simulink model "Grid_forming_reproduction"  (R2023b)
settings: Solver=VariableStepAuto  StartTime=0.0  StopTime=30  RelTol=1e-3
PreLoadFcn:
  | Ts = 50e-6;
InitFcn:
  | load Grid_forming_reproduction_Init
  | Ts = 50e-6;
undefined symbols (not defined in the file or in its folder): DiscIntNeverNeededParam, find_system
libraries: spsThreePhaseVIMeasurementLib x6, spsabctodq0Lib x6, slpidlib x4, spsThreePhaseSeriesRLCBranchLib x3, spsFirstOrderFilterLib x3, spsPower3phInstantaneousLib x3, simulink_extras x2, spsGroundLib x2, spsStairGeneratorLib x2, spsThreePhaseProgrammableVoltageSourceLib x1, spsdq0toabcLib x1, spsPLL3phLib x1
settings Model: Creator=DH7946  LastModifiedBy=DH7946
settings DataIOCC: LoadInitialState=on  SaveFormat=StructureWithTime  SaveOutput=off  SaveTime=off  ReturnWorkspaceOutputs=off
settings DebuggingCC: UnconnectedInputMsg=warning  UnconnectedOutputMsg=warning  UnconnectedLineMsg=warning
settings ModelReferenceCC: EnableRefExpFcnMdlSchedulingChecks=on
settings RTWCC: DLArmComputeVersion=19.05

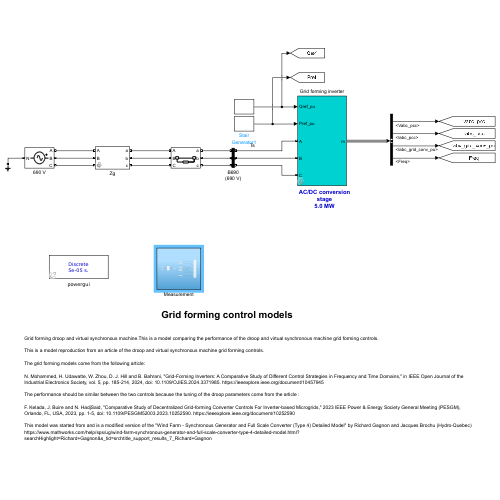
[thumbnail: Simulink's stored preview of the top-level diagram]
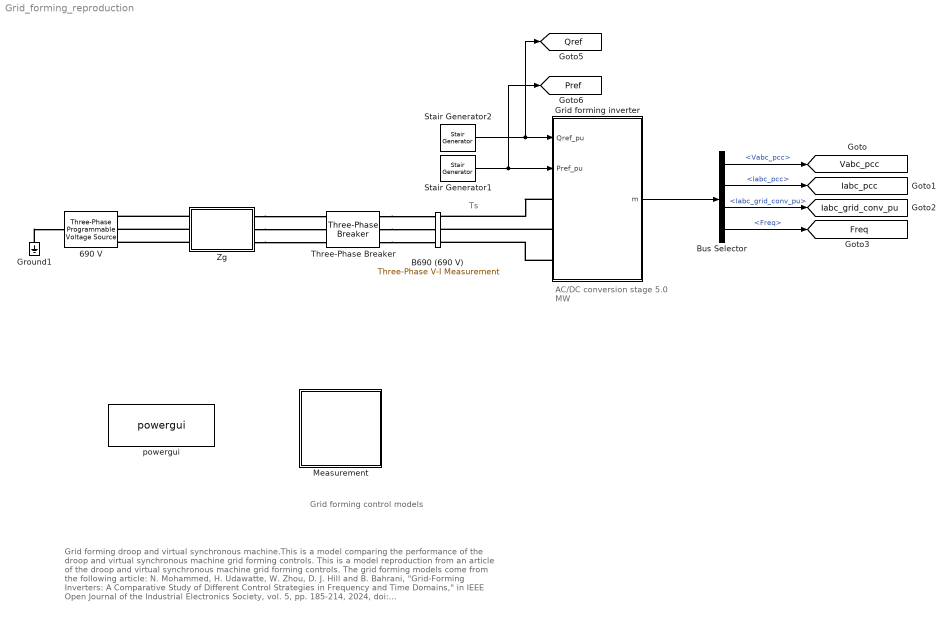
== system Grid_forming_reproduction ==
  note: Grid forming droop and virtual synchronous machine.This is a model comparing the performance of the droop and virtual synchronous machine grid forming controls.
      |
      | This is a model reproduction from an article of the droop and virtual synchronous machine grid forming controls.
      |
      | The grid forming models come from the following article:
      |
      | N. Mohammed, H. Udawatte, W. Zhou, D. J. Hill and B. Bahrani, "Grid-Forming Inverters: A Comparative Study of Different Control Strategies in Frequency and Time Domains," in IEEE Open Journal of the Industrial Electronics Society, vol. 5, pp. 185-214, 2024, doi: 10.1109/OJIES.2024.3371985. https://ieeexplore.ieee.org/document/10457945
      |
      | The performance should be similar between the two controls because the tuning of the droop parameters come from the article :
      |
      | F. Kelada, J. Buire and N. HadjSaid, "Comparative Study of Decentralized Grid-forming Converter Controls For Inverter-based Microgrids," 2023 IEEE Power & Energy Society General Meeting (PESGM), Orlando, FL, USA, 2023, pp. 1-5, doi: 10.1109/PESGM52003.2023.10252590. https://ieeexplore.ieee.org/document/10252590
      |
      | This model was started from and is a modified version of the "Wind Farm - Synchronous Generator and Full Scale Converter (Type 4) Detailed Model" by Richard Gagnon and Jacques Brochu (Hydro-Quebec)
      | https://www.mathworks.com/help/sps/ug/wind-farm-synchronous-generator-and-full-scale-converter-type-4-detailed-model.html?searchHighlight=Richard+Gagnon&s_tid=srchtitle_support_results_7_Richard+Gagnon
  note: Grid forming control models
  note: AC/DC conversion stage
      | 5.0 MW
  note: Ts
  690 V : spsThreePhaseProgrammableVoltageSourceLib/Three-Phase Programmable Voltage Source  PositiveSequence=[690 0 50]  VariationEntity=None  VariationType=Table of time-amplitude pairs  VariationTypeAlt=Step  VariationStep=-0.2  VariationRate=10  VariationMagnitude=0.3  VariationFrequency=2  VariationTiming=[5 6]  VariationPhaseA=off  Amplitudes=[1 0.75 1.0]  TimeValues=[0 50.03 50.13]  HarmonicGeneration=off  HarmonicA=[1 -0.1 0 2]  HarmonicB=[2 0.15 35 2]*0  Timing="[0.1  2]"  BusType=swing  Pref=0  Qref=0  Qmin=-inf  Qmax=inf
  B690 (690 V) : spsThreePhaseVIMeasurementLib/Three-Phase V-I Measurement  VoltageMeasurement=phase-to-ground  SetLabelV=on  LabelV=Vabc_B575  Vpu=off  VpuLL=off  CurrentMeasurement=yes  SetLabelI=on  LabelI=Iabc_B575  Ipu=off  Pbase=5*2e6/0.9  Vbase=575  OutputType=Complex  PhasorSimulation=off  PSBequivalent=0
  Bus Selector : BusSelector  OutputSignals=Vabc_pcc,Iabc_pcc,Iabc_grid_conv_pu,Freq
  Grid forming inverter : Subsystem  LoadFcn=%find_system(gcs,'FollowLinks', 'on', 'LookUnderMasks', 'all');  mask(Grid forming inverter){Vnom=690, fnom=50, Pnom=5e6, Lf=95e-6, Rf=10e-3, Cf=1e-3, Vdc_nom=2000, Innerloops=Inner loops, Kp_cc=0.1425, Ki_cc=15, Kffv=1, Kp_vc=14.25, Ki_vc=1500, Kffi=0.9, Virtualimpedance=Virtual impedance, Rvir=5e-3, Lvir=50e-6, ControlType=Droop, mp=0.7855e-6, nq=1.5e-5, Ki_q=1e-4, tau=0.001, Ts=Ts}
      mask prompts: Vnom "Grid-side converter nominal AC voltage (V):"; fnom "Grid frequency (Hz)"; Pnom "Nominal power (VA)"; Lf "Filter inductance (H)"; Rf "Filter resistance (Ω)"; Cf "Filter capacitor (F):"; Vdc_nom "Nominal DC bus voltage (V)"; Innerloops "Inner loops"; Kp_cc "Proportional gain of the current controller"; Ki_cc "Integral gain of the current controller"; Kffv "Voltage feed-forward"; Kp_vc "Proportional gain of the voltage controller"; Ki_vc "Integral gain of the voltage controller"; Kffi "Current feed-forward"; Virtualimpedance "Virtual impedance"; Rvir "Resistance of the virtual impedance"; Lvir "Inductance of the virtual impedance"; ControlType "Primary control"; mp "P - ω Droop coefficient"; nq "Q - V Droop coefficient"; Ki_q "Integral gain of the reactive power controller"; tau "Filter time constant (s)"; Ts "Sample time (s):"
      mask help: This block implements a model of a grid forming inverter with either droop or virtual synchronous generator control.
      mask init:
      | % Converters data
      | Q_filter=50;
      | 
      | % Controller data
      | Freq_filter=10000;   %Hz
      | Zeta_filter=0.707;
      | Mod_index_max=1.1;
      | T_speed=5;      %Speed reference time constant (s)
      | Iq_ref_limit_time_constant=0.3; %(s)
      | Current_reg_output_limit=1.1;   %(pu)
      | Var_reg_output_hi_limit=1.1;    %(pu)
      | Var_reg_output_low_limit=0.9;   %(pu)
      | Pitch_time_constant=0.01;       %(s)
      | Vf_limit=10;    %Field voltage limit (pu)
      | Freq_sawtooth=2000; %Hz, Boost converter
      | Freq_PWM=3000; %Hz, Inverter
      | Ts_snub=50e-6;  %Sample time to compute snubber resistance
      mask TypeOptions Innerloops: Inner loops | No inner loops
      mask Callback Innerloops:
      | BlockName=getfullname(gcb);
      | %
      | 
      | Param_Show=get_param(BlockName,'Innerloops');
      | p_mask=get_param(BlockName,'MaskVisibilities');
      | 
      | p_mask{8} = 'on';
      | 
      | p_mask{9}='off';p_mask{10}='off';p_mask{11}='off';p_mask{12}='off';
      | p_mask{13}='off';p_mask{14}='off';
      | 
      | p_mask{15} = 'on';
      | 
      | switch Param_Show
      |     case 'Inner loops'
      |         p_mask{9}='on';p_mask{10}='on';p_mask{11}='on';p_mask{12}='on';
      |         p_mask{13}='on';p_mask{14}='on';
      | 
      |     case 'No inner loops'
      | 
      | end
      | 
      | ParVisible=p_mask;
      | %
      | set_param(BlockName,'MaskVisibilities',ParVisible);
      mask TypeOptions Virtualimpedance: Virtual impedance | No virtual impedance
      mask Callback Virtualimpedance:
      | BlockName=getfullname(gcb);
      | %
      | Param_Show=get_param(BlockName,'Virtualimpedance');
      | p_mask=get_param(BlockName,'MaskVisibilities');
      | 
      | 
      | p_mask{16}='off';p_mask{17}='off';
      | 
      | 
      | 
      | switch Param_Show
      |     case 'Virtual impedance'
      |         p_mask{16}='on';p_mask{17}='on';
      | 
      |     case 'No virtual impedance'
      | 
      | end
      | 
      | ParVisible=p_mask;
      | %
      | set_param(BlockName,'MaskVisibilities',ParVisible);
      mask TypeOptions ControlType: Droop | Virtual Synchronous Machine
      mask Display: disp(' ');
  Ground1 : spsGroundLib/Ground  LConnTagsString=a
  Measurement : Subsystem
  Stair Generator1 : spsStairGeneratorLib/Stair Generator  t=[0, 10]  e=[2e6, 4e6]  Ts=0
  Stair Generator2 : spsStairGeneratorLib/Stair Generator  t=[0, 20]  e=[0, 3e6]  Ts=0
  Three-Phase Breaker : spsThreePhaseBreakerLib/Three-Phase Breaker  InitialState=closed  SwitchA=off  SwitchB=off  SwitchC=off  SwitchTimes="[1/60  5/60]"  External=off  BreakerResistance=1e-10  SnubberResistance=1e10  SnubberCapacitance=inf  Measurements=None
  Zg : Subsystem  mask{Pnom=5e6, SCR=1.5, XR=7, Vnom=690, fnom=50}
      mask prompts: Pnom "Nominal power (VA)"; SCR "Grid short circuit ratio"; XR "Grid X/R ratio"; Vnom "Grid-side converter nominal AC voltage (V):"; fnom "Grid frequency (Hz)"
  powergui : spspowerguiLib/powergui  SimulationMode=Discrete  SampleTime=Ts  frequency=60  Iterations=50  frequencyindice=0  Pbase=100e6  ErrMax=1e-4  UnitsV=kV  UnitsW=MW  buscounter=0  FunctionMessages=off  echomessages=off  EnableUseOfTLC=off  CurrentSourceSwitches=off  DisableSnubberDevices=off  DisableRonSwitches=off  DisableVfSwitches=off  DisplayEquations=off  AutomaticDiscreteSolvers=off  SolverType=Tustin  Interpol=off  ExternalGateDelay=off  methode=off  Ts=0  x0status=blocks  SPID=off  SwTol=0  HookPort=off  NonlinearTolerance=1e-4  nMaxIteration=100  ContinueOnMaxIteration=off  RestoreLinks=warning  ResistiveCurrentMeasurement=off  Frange=[0:2:500]  Ylog=off  Xlog=on  ShowGrid=off  save=off  variable=ZData  structure=0  ZoomFFT=on  StartTime=0.0  cycles=1  DisplayStyle=1  fundamental=60  FreqAxis=off  MaxFrequency=1000  frequencyindicesteady=1  RmsSteady=1  display=off
  tag scope: Freq=global, Iabc_grid_conv_pu=global, Iabc_pcc=global, Pref=global, Qref=global, Vabc_pcc=global
  wires:
  Stair Generator2/1 -> [Qref], Grid forming inverter/1(Qref_pu)
  Stair Generator1/1 -> [Pref], Grid forming inverter/2(Pref_pu)
  Grid forming inverter/1(m) -> Bus Selector/1
  Bus Selector/1 -> [Vabc_pcc]  "<Vabc_pcc>"
  Bus Selector/2 -> [Iabc_pcc]  "<Iabc_pcc>"
  Bus Selector/3 -> [Iabc_grid_conv_pu]  "<Iabc_grid_conv_pu>"
  Bus Selector/4 -> [Freq]  "<Freq>"
  connections:
  Three-Phase Breaker/RConn1 -- B690 (690 V)/LConn1
  Three-Phase Breaker/RConn2 -- B690 (690 V)/LConn2
  Three-Phase Breaker/RConn3 -- B690 (690 V)/LConn3
  Ground1/LConn1 -- 690 V/LConn1
  Grid forming inverter/LConn1 -- B690 (690 V)/RConn1
  Grid forming inverter/LConn2 -- B690 (690 V)/RConn2
  Grid forming inverter/LConn3 -- B690 (690 V)/RConn3
  Zg/LConn1 -- 690 V/RConn1
  Zg/RConn1 -- Three-Phase Breaker/LConn1
  Zg/LConn2 -- 690 V/RConn2
  Zg/RConn2 -- Three-Phase Breaker/LConn2
  Zg/LConn3 -- 690 V/RConn3
  Zg/RConn3 -- Three-Phase Breaker/LConn3

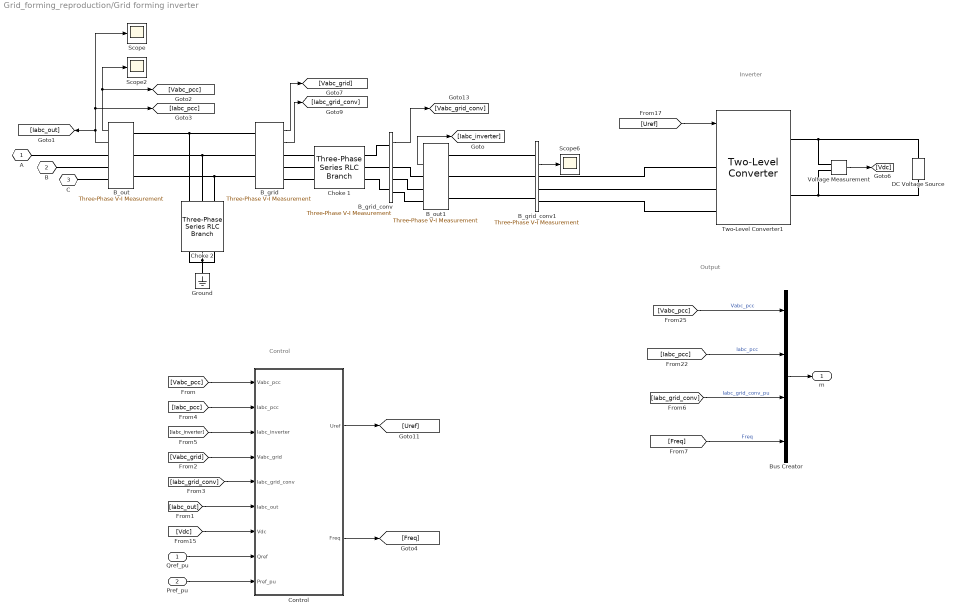
== system Grid_forming_reproduction/Grid forming inverter ==
  note: Control
  note: Inverter
  note: Output
  Qref_pu : Inport
  Pref_pu : Inport  Port=2
  B_grid : spsThreePhaseVIMeasurementLib/Three-Phase V-I Measurement  VoltageMeasurement=phase-to-ground  SetLabelV=off  LabelV=Vabc  Vpu=on  VpuLL=off  CurrentMeasurement=yes  SetLabelI=off  LabelI=Iabc  Ipu=on  Pbase=5e6  Vbase=690  OutputType=Complex  PhasorSimulation=off  PSBequivalent=0
  B_grid_conv : spsThreePhaseVIMeasurementLib/Three-Phase V-I Measurement  VoltageMeasurement=phase-to-ground  SetLabelV=off  LabelV=Vabc  Vpu=on  VpuLL=off  CurrentMeasurement=yes  SetLabelI=off  LabelI=Iabc  Ipu=off  Pbase=Pnom  Vbase=Vnom  OutputType=Complex  PhasorSimulation=off  PSBequivalent=0
  B_grid_conv1 : spsThreePhaseVIMeasurementLib/Three-Phase V-I Measurement  VoltageMeasurement=phase-to-ground  SetLabelV=off  LabelV=Vabc  Vpu=off  VpuLL=off  CurrentMeasurement=yes  SetLabelI=off  LabelI=Iabc  Ipu=off  Pbase=Pnom  Vbase=Vnom  OutputType=Complex  PhasorSimulation=off  PSBequivalent=0
  B_out : spsThreePhaseVIMeasurementLib/Three-Phase V-I Measurement  VoltageMeasurement=phase-to-ground  SetLabelV=off  LabelV=Vabc  Vpu=off  VpuLL=off  CurrentMeasurement=yes  SetLabelI=off  LabelI=Iabc  Ipu=off  Pbase=5e6  Vbase=690  OutputType=Complex  PhasorSimulation=off  PSBequivalent=0
  B_out1 : spsThreePhaseVIMeasurementLib/Three-Phase V-I Measurement  VoltageMeasurement=phase-to-ground  SetLabelV=off  LabelV=Vabc  Vpu=off  VpuLL=off  CurrentMeasurement=yes  SetLabelI=off  LabelI=Iabc  Ipu=off  Pbase=5e6  Vbase=690  OutputType=Complex  PhasorSimulation=off  PSBequivalent=0
  Bus Creator : BusCreator  Inputs=4
  Choke 1 : spsThreePhaseSeriesRLCBranchLib/Three-Phase Series RLC Branch  LConnTagsString=A|B|C  RConnTagsString=A|B|C  BranchType=RL  Resistance=Rf  Inductance=Lf  Capacitance=[]  Measurements=None
  Choke 2 : spsThreePhaseSeriesRLCBranchLib/Three-Phase Series RLC Branch  LConnTagsString=A|B|C  RConnTagsString=A|B|C  BranchType=C  Resistance=10e-3  Inductance=95e-6  Capacitance=Cf  Measurements=None
  Control : Subsystem
  DC Voltage Source : spsDCVoltageSourceLib/DC Voltage Source  Amplitude=Vdc_nom  Measurements=None
  Ground : spsGroundLib/Ground  LConnTagsString=a
  Scope : Scope
  Scope2 : Scope
  Scope6 : Scope
  Two-Level Converter1 : spsTwoLevelConverterLib/Two-Level Converter  ModelType=Average model (Uref-controlled)  Ron=1e-3  Rs=1e6  Cs=inf  Vforward=[0,0]  Ron_Diode=1e-3  Rs_Diode=1e6  Cs_Diode=inf  Vf_Diode=1e-3  Rs_CurrentSource=inf  Ron_ACsource=1e-3
  Voltage Measurement : spsVoltageMeasurementLib/Voltage Measurement  PhasorSimulation=off  OutputType=Complex  PSBequivalent=0
  A : PMIOPort  Tag=PMCPort  Side=Left
  B : PMIOPort  Tag=PMCPort  Port=2  Side=Left
  C : PMIOPort  Tag=PMCPort  Port=3  Side=Left
  m : Outport  VectorParamsAs1DForOutWhenUnconnected=off
  wires:
  B_grid_conv/1 -> [Vabc_grid_conv]
  B_grid/1 -> [Vabc_grid]
  B_grid/2 -> [Iabc_grid_conv]
  [Vabc_grid] -> Control/4(Vabc_grid)
  [Iabc_grid_conv] -> Control/5(Iabc_grid_conv)
  [Vdc] -> Control/7(Vdc)
  Qref_pu/1 -> Control/8(Qref)
  Control/1(Uref) -> [Uref]
  [Uref] -> Two-Level Converter1/1
  [Vabc_pcc] -> Bus Creator/1  "Vabc_pcc"
  Bus Creator/1 -> m/1
  [Iabc_pcc] -> Bus Creator/2  "Iabc_pcc"
  [Iabc_grid_conv] -> Bus Creator/3  "Iabc_grid_conv_pu"
  [Iabc_out] -> Control/6(Iabc_out)
  Pref_pu/1 -> Control/9(Pref_pu)
  Voltage Measurement/1 -> [Vdc]
  B_out/1 -> [Vabc_pcc], Scope2/1
  [Vabc_pcc] -> Control/1(Vabc_pcc)
  [Iabc_pcc] -> Control/2(Iabc_pcc)
  [Iabc_inverter] -> Control/3(Iabc_inverter)
  B_out1/2 -> [Iabc_inverter]
  B_grid_conv1/2 -> Scope6/1
  B_out/2 -> Scope/1, [Iabc_pcc], [Iabc_out]
  Control/2(Freq) -> [Freq]
  [Freq] -> Bus Creator/4  "Freq"
  connections:
  B_out/LConn1 -- Choke 2/LConn1 -- B_grid/LConn1
  B_out/LConn2 -- Choke 2/LConn2 -- B_grid/LConn2
  B_out/LConn3 -- Choke 2/LConn3 -- B_grid/LConn3
  Voltage Measurement/LConn2 -- DC Voltage Source/LConn1 -- Two-Level Converter1/RConn2
  Voltage Measurement/LConn1 -- DC Voltage Source/RConn1 -- Two-Level Converter1/RConn1
  C/RConn1 -- B_out/RConn3
  B_out/RConn2 -- B/RConn1
  A/RConn1 -- B_out/RConn1
  Two-Level Converter1/LConn1 -- B_grid_conv1/RConn1
  B_grid_conv1/RConn2 -- Two-Level Converter1/LConn2
  B_grid_conv1/RConn3 -- Two-Level Converter1/LConn3
  B_out1/LConn1 -- B_grid_conv1/LConn1
  B_out1/LConn3 -- B_grid_conv1/LConn3
  Choke 2/RConn2 -- Ground/LConn1 -- Choke 2/RConn1 -- Choke 2/RConn3
  B_grid_conv1/LConn2 -- B_out1/LConn2
  B_out1/RConn1 -- B_grid_conv/RConn1
  B_out1/RConn2 -- B_grid_conv/RConn2
  B_out1/RConn3 -- B_grid_conv/RConn3
  Choke 1/RConn2 -- B_grid_conv/LConn2
  B_grid_conv/LConn1 -- Choke 1/RConn1
  B_grid_conv/LConn3 -- Choke 1/RConn3
  Choke 1/LConn1 -- B_grid/RConn1
  Choke 1/LConn2 -- B_grid/RConn2
  Choke 1/LConn3 -- B_grid/RConn3

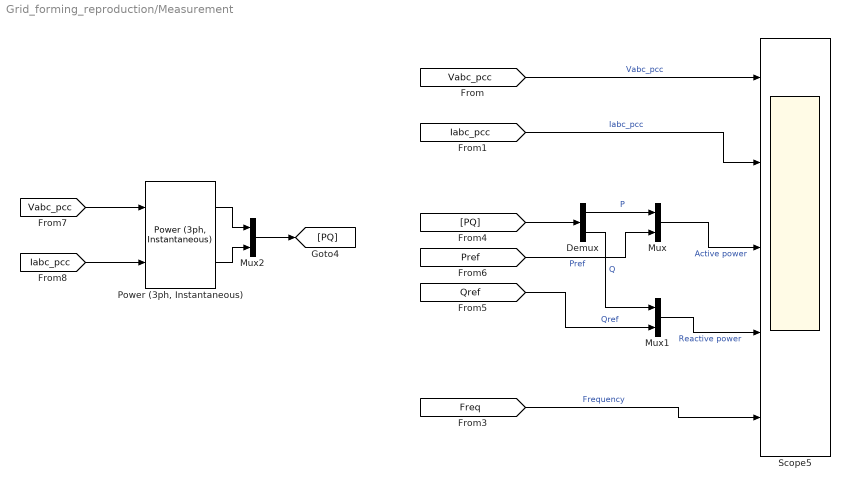
== system Grid_forming_reproduction/Measurement ==
  Demux : Demux  Outputs=2
  Mux : Mux  Inputs=2
  Mux1 : Mux  Inputs=2
  Mux2 : Mux  Inputs=2
  "Power (3ph, Instantaneous)" : spsPower3phInstantaneousLib/Power (3ph, Instantaneous)
  Scope5 : Scope  NumInputPorts=5
  wires:
  [PQ] -> Demux/1
  [Pref] -> Mux/2  "Pref"
  Demux/1 -> Mux/1  "P"
  Demux/2 -> Mux1/1  "Q"
  [Qref] -> Mux1/2  "Qref"
  Mux1/1 -> Scope5/4  "Reactive power"
  Mux/1 -> Scope5/3  "Active power"
  "Power (3ph, Instantaneous)"/2 -> Mux2/2
  [Vabc_pcc] -> "Power (3ph, Instantaneous)"/1
  [Iabc_pcc] -> "Power (3ph, Instantaneous)"/2
  "Power (3ph, Instantaneous)"/1 -> Mux2/1
  Mux2/1 -> [PQ]
  [Freq] -> Scope5/5  "Frequency"
  [Vabc_pcc] -> Scope5/1  "Vabc_pcc"
  [Iabc_pcc] -> Scope5/2  "Iabc_pcc"

== system Grid_forming_reproduction/Zg ==
  Three-Phase Series RLC Branch : spsThreePhaseSeriesRLCBranchLib/Three-Phase Series RLC Branch  LConnTagsString=A|B|C  RConnTagsString=A|B|C  BranchType=RL  Resistance=(2*pi*fnom*(((Vnom^2)/(SCR*Pnom))/(2*pi*fnom)))/XR  Inductance=((Vnom^2)/(SCR*Pnom))/(2*pi*fnom)  Capacitance=1e-6  Measurements=None
  A : PMIOPort  Side=Left
  a : PMIOPort  Port=2  Side=Right
  B : PMIOPort  Port=3  Side=Left
  b : PMIOPort  Port=4  Side=Right
  C : PMIOPort  Port=5  Side=Left
  c : PMIOPort  Port=6  Side=Right
  connections:
  Three-Phase Series RLC Branch/LConn2 -- B/RConn1
  Three-Phase Series RLC Branch/RConn1 -- a/RConn1
  Three-Phase Series RLC Branch/RConn3 -- c/RConn1
  Three-Phase Series RLC Branch/LConn1 -- A/RConn1
  Three-Phase Series RLC Branch/LConn3 -- C/RConn1
  Three-Phase Series RLC Branch/RConn2 -- b/RConn1

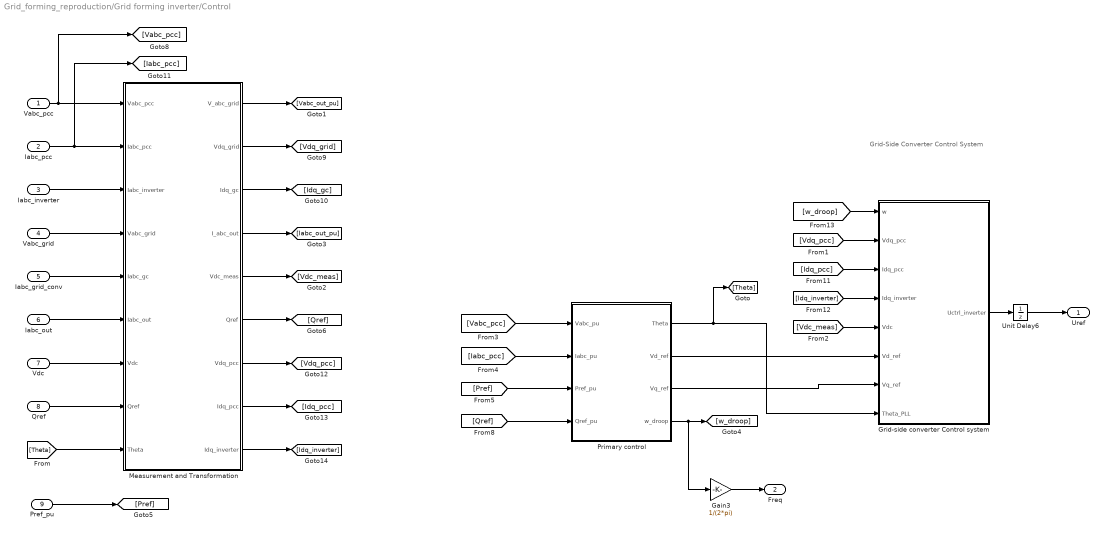
== system Grid_forming_reproduction/Grid forming inverter/Control ==
  note: Grid-Side Converter
      | Control System
  Vabc_pcc : Inport
  Iabc_pcc : Inport  Port=2
  Iabc_inverter : Inport  Port=3
  Vabc_grid : Inport  Port=4
  Iabc_grid_conv : Inport  Port=5
  Iabc_out : Inport  Port=6
  Vdc : Inport  Port=7
  Qref : Inport  Port=8
  Pref_pu : Inport  Port=9
  Gain3 : Gain  Gain=1/(2*pi)
  Grid-side converter Control system : Subsystem
  Measurement and Transformation : Subsystem
  Primary control : Subsystem  Variant=on  VariantControl=Choice
  Unit Delay6 : UnitDelay  SampleTime=Ts  HasFrameUpgradeWarning=on
  Uref : Outport  VectorParamsAs1DForOutWhenUnconnected=off
  Freq : Outport  Port=2  VectorParamsAs1DForOutWhenUnconnected=off
  wires:
  [Vdq_pcc] -> Grid-side converter Control system/2(Vdq_pcc)
  [Vdc_meas] -> Grid-side converter Control system/5(Vdc)
  Grid-side converter Control system/1(Uctrl_inverter) -> Unit Delay6/1
  Unit Delay6/1 -> Uref/1
  Vabc_grid/1 -> Measurement and Transformation/4(Vabc_grid)
  Iabc_grid_conv/1 -> Measurement and Transformation/5(Iabc_gc)
  Vdc/1 -> Measurement and Transformation/7(Vdc)
  Qref/1 -> Measurement and Transformation/8(Qref)
  Measurement and Transformation/2(Vdq_grid) -> [Vdq_grid]
  Measurement and Transformation/3(Idq_gc) -> [Idq_gc]
  Measurement and Transformation/5(Vdc_meas) -> [Vdc_meas]
  Measurement and Transformation/6("Qref ") -> [Qref]
  Iabc_out/1 -> Measurement and Transformation/6(Iabc_out)
  [Theta] -> Measurement and Transformation/9(Theta)
  Measurement and Transformation/4(I_abc_out) -> [Iabc_out_pu]
  Measurement and Transformation/1(V_abc_grid) -> [Vabc_out_pu]
  Pref_pu/1 -> [Pref]
  Vabc_pcc/1 -> [Vabc_pcc], Measurement and Transformation/1(Vabc_pcc)
  Iabc_pcc/1 -> [Iabc_pcc], Measurement and Transformation/2(Iabc_pcc)
  Iabc_inverter/1 -> Measurement and Transformation/3(Iabc_inverter)
  [Idq_pcc] -> Grid-side converter Control system/3(Idq_pcc)
  [Idq_inverter] -> Grid-side converter Control system/4(Idq_inverter)
  Measurement and Transformation/7(Vdq_pcc) -> [Vdq_pcc]
  Measurement and Transformation/8(Idq_pcc) -> [Idq_pcc]
  Measurement and Transformation/9(Idq_inverter) -> [Idq_inverter]
  [w_droop] -> Grid-side converter Control system/1(w)
  [Vabc_pcc] -> Primary control/1(Vabc_pu)
  [Iabc_pcc] -> Primary control/2(Iabc_pu)
  [Pref] -> Primary control/3(Pref_pu)
  [Qref] -> Primary control/4(Qref_pu)
  Primary control/1(Theta) -> Grid-side converter Control system/8(Theta_PLL), [Theta]
  Primary control/2(Vd_ref) -> Grid-side converter Control system/6(Vd_ref)
  Primary control/3(Vq_ref) -> Grid-side converter Control system/7(Vq_ref)
  Primary control/4(w_droop) -> Gain3/1, [w_droop]
  Gain3/1 -> Freq/1

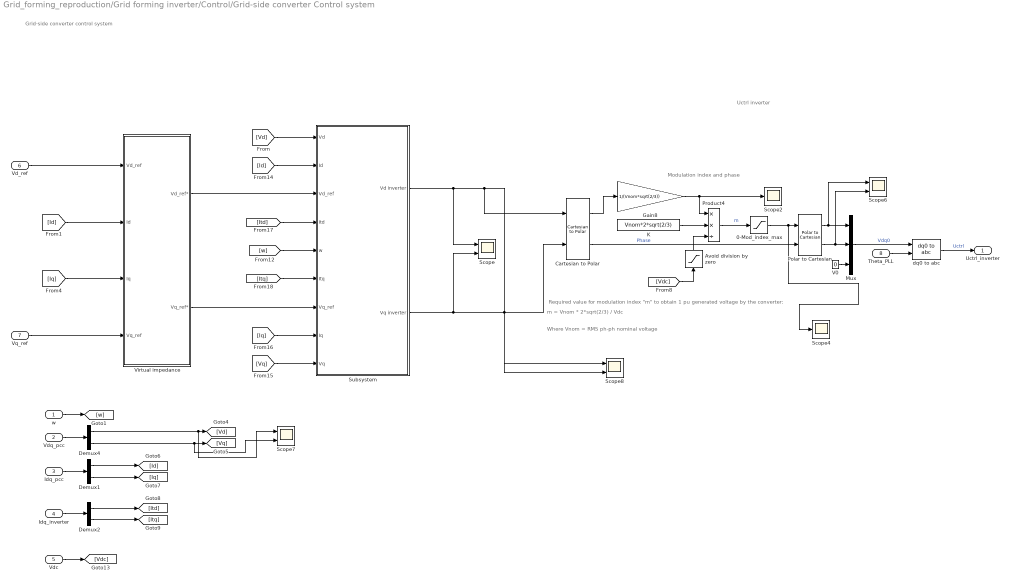
== system Grid_forming_reproduction/Grid forming inverter/Control/Grid-side converter Control system ==
  note: Modulation index and phase
  note: Where Vnom = RMS ph-ph nominal voltage
  note: m = Vnom * 2*sqrt(2/3) / Vdc
  note: Required value for modulation index "m" to obtain 1 pu generated voltage by the converter:
  note: Grid-side converter control system
  note: Uctrl inverter
  w : Inport
  Vdq_pcc : Inport  Port=2
  Idq_pcc : Inport  Port=3
  Idq_inverter : Inport  Port=4
  Vdc : Inport  Port=5
  Vd_ref : Inport  Port=6
  Vq_ref : Inport  Port=7
  Theta_PLL : Inport  Port=8
  0-Mod_index_max : Saturate  UpperLimit=Mod_index_max*0+1.4  LowerLimit=0
  Avoid division by zero : Saturate  UpperLimit=1e6  LowerLimit=1e-6
  Cartesian to Polar : simulink_extras/Transformations/Cartesian to Polar
  Demux1 : Demux  Outputs=2
      settings: DisplayOption=none
  Demux2 : Demux  Outputs=2
      settings: DisplayOption=none
  Demux4 : Demux  Outputs=2
      settings: DisplayOption=none
  Gain8 : Gain  Gain=1/(Vnom*sqrt(2/3))
  K : Constant  Value=Vnom*2*sqrt(2/3)
  Mux : Mux  Inputs=3
  Polar to Cartesian : simulink_extras/Transformations/Polar to Cartesian
  Product4 : Product  Inputs=**/  InputSameDT=on  SaturateOnIntegerOverflow=on  OutDataTypeStr=Inherit: Same as first input
  Scope{,6..8} (4 alike) : Scope  NumInputPorts=2
  Scope2 : Scope
  Scope4 : Scope
  Subsystem : Subsystem  Variant=on  VariantControl=Choice
  V0 : Constant  Value=0
  Virtual impedance : Subsystem  Variant=on  VariantControl=Choice
  dq0 to abc : spsdq0toabcLib/dq0 to abc  Alignment=90 degrees behind phase A axis
  Uctrl_inverter : Outport  VectorParamsAs1DForOutWhenUnconnected=off
  wires:
  0-Mod_index_max/1 -> Polar to Cartesian/1, Scope4/1
  Cartesian to Polar/2 -> Polar to Cartesian/2  "Phase"
  [Vdc] -> Avoid division by zero/1
  Cartesian to Polar/1 -> Gain8/1
  Avoid division by zero/1 -> Product4/3
  K/1 -> Product4/2
  Product4/1 -> 0-Mod_index_max/1  "m"
  Demux4/2 -> Scope7/2, [Vq]
  Demux4/1 -> Scope7/1, [Vd]
  w/1 -> [w]
  Vdq_pcc/1 -> Demux4/1
  Vdc/1 -> [Vdc]
  Idq_pcc/1 -> Demux1/1
  Demux1/1 -> [Id]
  Demux1/2 -> [Iq]
  Demux2/2 -> [Itq]
  Demux2/1 -> [Itd]
  Idq_inverter/1 -> Demux2/1
  Polar to Cartesian/1 -> Mux/1, Scope6/1
  Theta_PLL/1 -> dq0 to abc/2
  V0/1 -> Mux/3
  Polar to Cartesian/2 -> Mux/2, Scope6/2
  Mux/1 -> dq0 to abc/1  "Vdq0"
  dq0 to abc/1 -> Uctrl_inverter/1  "Uctrl"
  Gain8/1 -> Product4/1, Scope2/1
  Vd_ref/1 -> Virtual impedance/1(Vd_ref)
  [Id] -> Virtual impedance/2(Id)
  [Iq] -> Virtual impedance/3(Iq)
  Vq_ref/1 -> Virtual impedance/4(Vq_ref)
  Subsystem/1(Vd inverter) -> Scope/1, Scope8/1, Cartesian to Polar/1
  Subsystem/2(Vq inverter) -> Scope/2, Cartesian to Polar/2, Scope8/2
  [Vd] -> Subsystem/1(Vd)
  [Id] -> Subsystem/2(Id)
  [Vq] -> Subsystem/9(Vq)
  Virtual impedance/1(Vd_ref*) -> Subsystem/3(Vd_ref)
  [Iq] -> Subsystem/8(Iq)
  [Itd] -> Subsystem/4(Itd)
  Virtual impedance/2(Vq_ref*) -> Subsystem/7(Vq_ref)
  [w] -> Subsystem/5(w)
  [Itq] -> Subsystem/6(Itq)

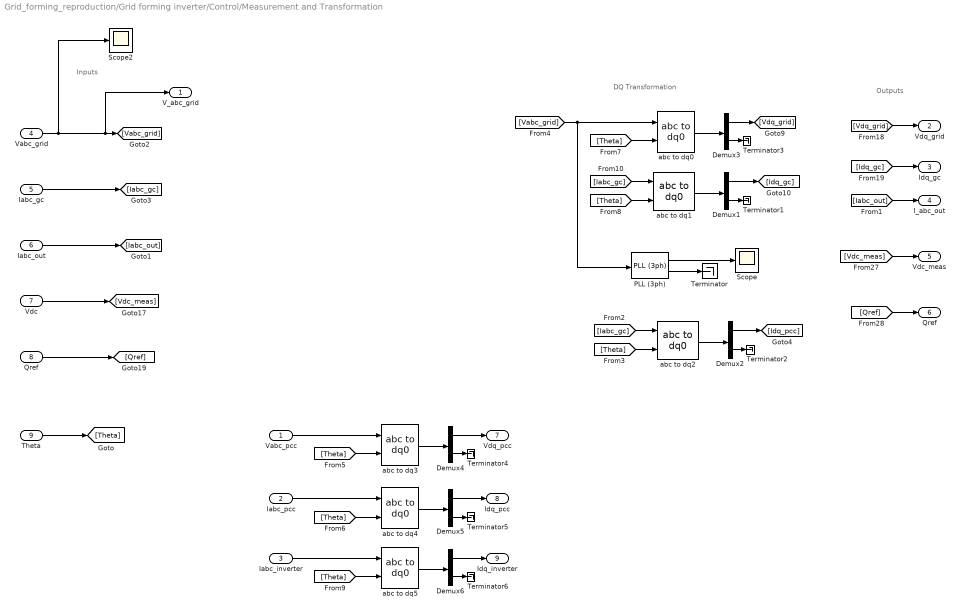
== system Grid_forming_reproduction/Grid forming inverter/Control/Measurement and Transformation ==
  note: Inputs
  note: DQ Transformation
  note: Outputs
  Vabc_pcc : Inport
  Iabc_pcc : Inport  Port=2
  Iabc_inverter : Inport  Port=3
  Vabc_grid : Inport  Port=4
  Iabc_gc : Inport  Port=5
  Iabc_out : Inport  Port=6
  Vdc : Inport  Port=7
  Qref : Inport  Port=8
  Theta : Inport  Port=9
  Demux{1..6} (6 alike) : Demux  Outputs=[2 1]
      settings: DisplayOption=none
  PLL (3ph) : spsPLL3phLib/PLL (3ph)  Fmin=35  Par_Init=[0, 50]  ParK=[180, 3200, 0]  TcD=1e-4  MaxRateChangeFreq=12  FilterCutOffFreq=25  Ts=Ts  AGC=on
  Scope : Scope
  Scope2 : Scope
  Terminator{,1..6} (7 alike) : Terminator
  abc to dq{0..5} (6 alike) : spsabctodq0Lib/abc to dq0  Alignment=90 degrees behind phase A axis
  V_abc_grid : Outport  VectorParamsAs1DForOutWhenUnconnected=off
  Vdq_grid : Outport  Port=2  VectorParamsAs1DForOutWhenUnconnected=off
  Idq_gc : Outport  Port=3  VectorParamsAs1DForOutWhenUnconnected=off
  I_abc_out : Outport  Port=4  VectorParamsAs1DForOutWhenUnconnected=off
  Vdc_meas : Outport  Port=5  VectorParamsAs1DForOutWhenUnconnected=off
  "Qref " : Outport  Port=6  VectorParamsAs1DForOutWhenUnconnected=off
  Vdq_pcc : Outport  Port=7  VectorParamsAs1DForOutWhenUnconnected=off
  Idq_pcc : Outport  Port=8  VectorParamsAs1DForOutWhenUnconnected=off
  Idq_inverter : Outport  Port=9  VectorParamsAs1DForOutWhenUnconnected=off
  wires:
  Qref/1 -> [Qref]
  Vdc/1 -> [Vdc_meas]
  Iabc_gc/1 -> [Iabc_gc]
  Vabc_grid/1 -> V_abc_grid/1, [Vabc_grid], Scope2/1
  [Qref] -> "Qref "/1
  [Vdc_meas] -> Vdc_meas/1
  [Idq_gc] -> Idq_gc/1
  [Vdq_grid] -> Vdq_grid/1
  Demux1/1 -> [Idq_gc]
  [Iabc_gc] -> abc to dq1/1
  [Theta] -> abc to dq1/2
  [Vabc_grid] -> PLL (3ph)/1, abc to dq0/1
  abc to dq0/1 -> Demux3/1
  abc to dq1/1 -> Demux1/1
  Demux3/2 -> Terminator3/1
  Demux3/1 -> [Vdq_grid]
  Demux1/2 -> Terminator1/1
  Theta/1 -> [Theta]
  Iabc_out/1 -> [Iabc_out]
  [Iabc_out] -> I_abc_out/1
  PLL (3ph)/2 -> Terminator/1
  PLL (3ph)/1 -> Scope/1
  [Theta] -> abc to dq0/2
  Demux2/1 -> [Idq_pcc]
  abc to dq2/1 -> Demux2/1
  [Theta] -> abc to dq2/2
  Demux2/2 -> Terminator2/1
  [Iabc_gc] -> abc to dq2/1
  abc to dq3/1 -> Demux4/1
  [Theta] -> abc to dq3/2
  Demux4/2 -> Terminator4/1
  Demux4/1 -> Vdq_pcc/1
  [Theta] -> abc to dq4/2
  Demux5/2 -> Terminator5/1
  Demux5/1 -> Idq_pcc/1
  abc to dq4/1 -> Demux5/1
  Demux6/2 -> Terminator6/1
  abc to dq5/1 -> Demux6/1
  Demux6/1 -> Idq_inverter/1
  [Theta] -> abc to dq5/2
  Vabc_pcc/1 -> abc to dq3/1
  Iabc_pcc/1 -> abc to dq4/1
  Iabc_inverter/1 -> abc to dq5/1

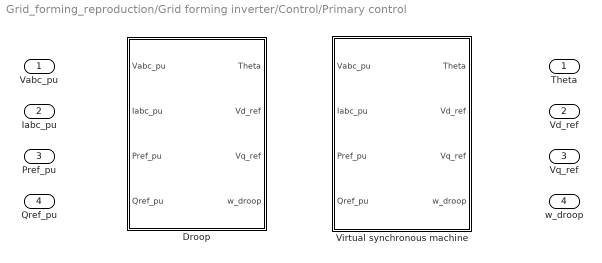
== system Grid_forming_reproduction/Grid forming inverter/Control/Primary control ==
  Vabc_pu : Inport
  Iabc_pu : Inport  Port=2
  Pref_pu : Inport  Port=3
  Qref_pu : Inport  Port=4
  Droop : Subsystem  VariantControl=ControlType == 1
  Virtual synchronous machine : Subsystem  VariantControl=ControlType == 2
  Theta : Outport
  Vd_ref : Outport  Port=2
  Vq_ref : Outport  Port=3
  w_droop : Outport  Port=4

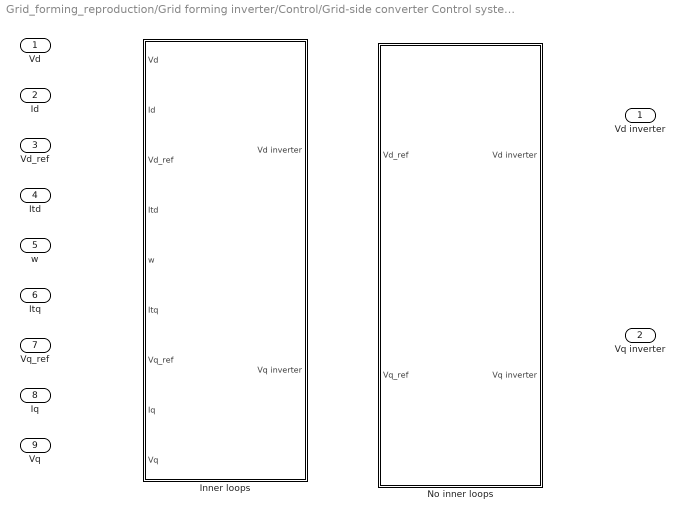
== system Grid_forming_reproduction/Grid forming inverter/Control/Grid-side converter Control system/Subsystem ==
  Vd : Inport
  Id : Inport  Port=2
  Vd_ref : Inport  Port=3
  Itd : Inport  Port=4
  w : Inport  Port=5
  Itq : Inport  Port=6
  Vq_ref : Inport  Port=7
  Iq : Inport  Port=8
  Vq : Inport  Port=9
  Inner loops : Subsystem  VariantControl=Innerloops == 1
  No inner loops : Subsystem  VariantControl=Innerloops == 2
  Vd inverter : Outport
  Vq inverter : Outport  Port=2

== system Grid_forming_reproduction/Grid forming inverter/Control/Grid-side converter Control system/Virtual impedance ==
  Vd_ref : Inport
  Id : Inport  Port=2
  Iq : Inport  Port=3
  Vq_ref : Inport  Port=4
  No virtual impedance : Subsystem  VariantControl=Virtualimpedance == 2
  Virtual impedance : Subsystem  VariantControl=Virtualimpedance == 1
  Vd_ref* : Outport
  Vq_ref* : Outport  Port=2

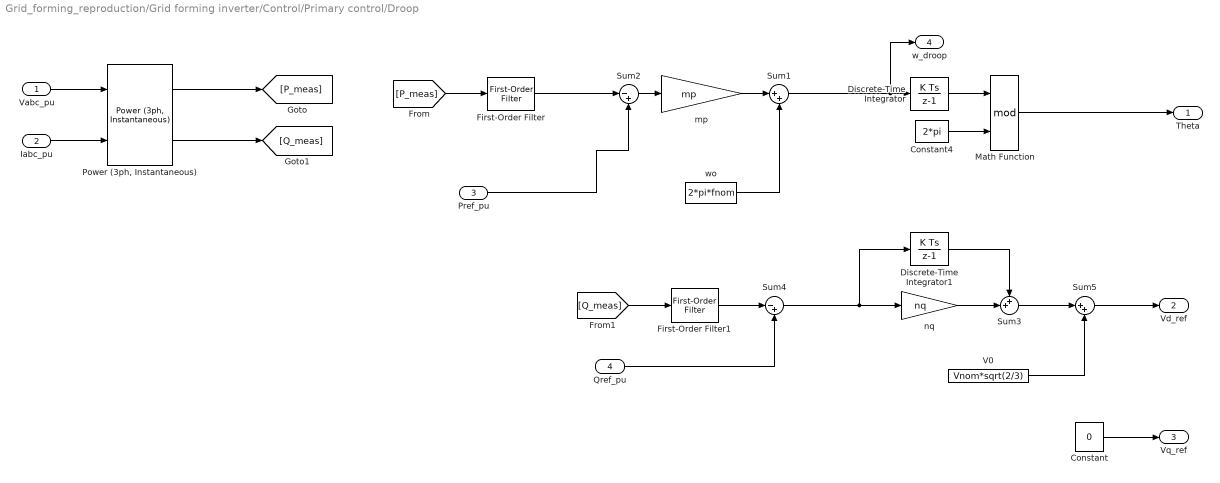
== system Grid_forming_reproduction/Grid forming inverter/Control/Primary control/Droop ==
  Vabc_pu : Inport
  Iabc_pu : Inport  Port=2
  Pref_pu : Inport  Port=3
  Qref_pu : Inport  Port=4
  Constant : Constant  Value=0
  Constant4 : Constant  Value=2*pi
  Discrete-Time Integrator : DiscreteIntegrator  gainval=1  SampleTime=Ts  ICPrevOutput=DiscIntNeverNeededParam  ICPrevScaledInput=DiscIntNeverNeededParam
  Discrete-Time Integrator1 : DiscreteIntegrator  gainval=Ki_q  SampleTime=Ts  ICPrevOutput=DiscIntNeverNeededParam  ICPrevScaledInput=DiscIntNeverNeededParam
  First-Order Filter : spsFirstOrderFilterLib/First-Order Filter  FilterType=Lowpass  Tc=tau  Ts=Ts  Initialize=off  Vac_Init=[0, 0, 60]  Vdc_Init=0  PlotResponse=off  FreqRange="[0,  200,  1]"
  First-Order Filter1 : spsFirstOrderFilterLib/First-Order Filter  FilterType=Lowpass  Tc=tau  Ts=Ts  Initialize=off  Vac_Init=[0, 0, 60]  Vdc_Init=0  PlotResponse=off  FreqRange="[0,  200,  1]"
  Math Function : Math  Operator=mod  SignedPower=on
  "Power (3ph, Instantaneous)" : spsPower3phInstantaneousLib/Power (3ph, Instantaneous)
  Sum1 : Sum  Inputs=|++  InputSameDT=on  SaturateOnIntegerOverflow=on  OutDataTypeStr=Inherit: Same as first input
  Sum2 : Sum  Inputs=|-+  InputSameDT=on  SaturateOnIntegerOverflow=on  OutDataTypeStr=Inherit: Same as first input
  Sum3 : Sum  Inputs=++|  InputSameDT=on  SaturateOnIntegerOverflow=on  OutDataTypeStr=Inherit: Same as first input
  Sum4 : Sum  Inputs=|-+  InputSameDT=on  SaturateOnIntegerOverflow=on  OutDataTypeStr=Inherit: Same as first input
  Sum5 : Sum  Inputs=|++  InputSameDT=on  SaturateOnIntegerOverflow=on  OutDataTypeStr=Inherit: Same as first input
  V0 : Constant  Value=Vnom*sqrt(2/3)
  mp : Gain  Gain=mp
  nq : Gain  Gain=nq
  wo : Constant  Value=2*pi*fnom
  Theta : Outport
  Vd_ref : Outport  Port=2
  Vq_ref : Outport  Port=3
  w_droop : Outport  Port=4
  wires:
  Constant4/1 -> Math Function/2
  Discrete-Time Integrator/1 -> Math Function/1
  wo/1 -> Sum1/2
  mp/1 -> Sum1/1
  Sum2/1 -> mp/1
  First-Order Filter/1 -> Sum2/1
  Pref_pu/1 -> Sum2/2
  Vabc_pu/1 -> "Power (3ph, Instantaneous)"/1
  Iabc_pu/1 -> "Power (3ph, Instantaneous)"/2
  "Power (3ph, Instantaneous)"/1 -> [P_meas]
  "Power (3ph, Instantaneous)"/2 -> [Q_meas]
  [P_meas] -> First-Order Filter/1
  Constant/1 -> Vq_ref/1
  Sum3/1 -> Sum5/1
  V0/1 -> Sum5/2
  nq/1 -> Sum3/2
  Sum4/1 -> Discrete-Time Integrator1/1, nq/1
  [Q_meas] -> First-Order Filter1/1
  First-Order Filter1/1 -> Sum4/1
  Qref_pu/1 -> Sum4/2
  Sum1/1 -> w_droop/1, Discrete-Time Integrator/1
  Math Function/1 -> Theta/1
  Discrete-Time Integrator1/1 -> Sum3/1
  Sum5/1 -> Vd_ref/1

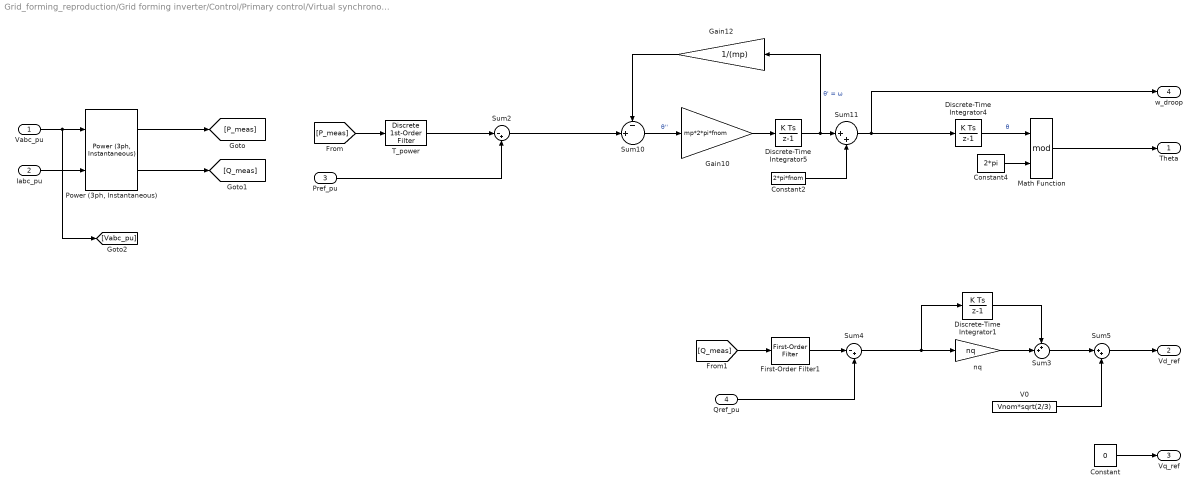
== system Grid_forming_reproduction/Grid forming inverter/Control/Primary control/Virtual synchronous machine ==
  Vabc_pu : Inport
  Iabc_pu : Inport  Port=2
  Pref_pu : Inport  Port=3
  Qref_pu : Inport  Port=4
  Constant : Constant  Value=0
  Constant2 : Constant  Value=2*pi*fnom
  Constant4 : Constant  Value=2*pi
  Discrete-Time Integrator1 : DiscreteIntegrator  gainval=Ki_q  SampleTime=Ts  ICPrevOutput=DiscIntNeverNeededParam  ICPrevScaledInput=DiscIntNeverNeededParam
  Discrete-Time Integrator4 : DiscreteIntegrator  SampleTime=-1  ICPrevOutput=DiscIntNeverNeededParam  ICPrevScaledInput=DiscIntNeverNeededParam
  Discrete-Time Integrator5 : DiscreteIntegrator  SampleTime=-1  ICPrevOutput=DiscIntNeverNeededParam  ICPrevScaledInput=DiscIntNeverNeededParam
  First-Order Filter1 : spsFirstOrderFilterLib/First-Order Filter  FilterType=Lowpass  Tc=tau  Ts=Ts  Initialize=off  Vac_Init=[0, 0, 60]  Vdc_Init=0  PlotResponse=off  FreqRange="[0,  200,  1]"
  Gain10 : Gain  Gain=mp*2*pi*fnom
  Gain12 : Gain  Gain=1/(mp)
  Math Function : Math  Operator=mod  SignedPower=on
  "Power (3ph, Instantaneous)" : spsPower3phInstantaneousLib/Power (3ph, Instantaneous)
  Sum10 : Sum  Inputs=-|+||
  Sum11 : Sum  Inputs=|++
  Sum2 : Sum  Inputs=|-+  InputSameDT=on  SaturateOnIntegerOverflow=on  OutDataTypeStr=Inherit: Same as first input
  Sum3 : Sum  Inputs=++|  InputSameDT=on  SaturateOnIntegerOverflow=on  OutDataTypeStr=Inherit: Same as first input
  Sum4 : Sum  Inputs=|-+  InputSameDT=on  SaturateOnIntegerOverflow=on  OutDataTypeStr=Inherit: Same as first input
  Sum5 : Sum  Inputs=|++  InputSameDT=on  SaturateOnIntegerOverflow=on  OutDataTypeStr=Inherit: Same as first input
  T_power : powerlib_extras/Discrete  Control Blocks/Discrete 1st-Order Filter  FilterType=Lowpass  Tc=tau  Ts=Ts  Initialize=on  Vac_Init=[0 0 0]  Vdc_Init=1  PlotResponse=off  param1=[1 500 0.1]
  V0 : Constant  Value=Vnom*sqrt(2/3)
  nq : Gain  Gain=nq
  Theta : Outport
  Vd_ref : Outport  Port=2
  Vq_ref : Outport  Port=3
  w_droop : Outport  Port=4
  wires:
  Constant4/1 -> Math Function/2
  T_power/1 -> Sum2/1
  Pref_pu/1 -> Sum2/2
  Vabc_pu/1 -> [Vabc_pu], "Power (3ph, Instantaneous)"/1
  Iabc_pu/1 -> "Power (3ph, Instantaneous)"/2
  "Power (3ph, Instantaneous)"/1 -> [P_meas]
  "Power (3ph, Instantaneous)"/2 -> [Q_meas]
  [P_meas] -> T_power/1
  Math Function/1 -> Theta/1
  Discrete-Time Integrator5/1 -> Sum11/1, Gain12/1  "θ' = ω"
  Sum2/1 -> Sum10/2
  Discrete-Time Integrator4/1 -> Math Function/1  "θ"
  Sum10/1 -> Gain10/1  "θ''"
  Gain10/1 -> Discrete-Time Integrator5/1
  Gain12/1 -> Sum10/1
  Sum11/1 -> Discrete-Time Integrator4/1, w_droop/1
  Constant2/1 -> Sum11/2
  Sum3/1 -> Sum5/1
  nq/1 -> Sum3/2
  Discrete-Time Integrator1/1 -> Sum3/1
  Sum4/1 -> Discrete-Time Integrator1/1, nq/1
  First-Order Filter1/1 -> Sum4/1
  V0/1 -> Sum5/2
  [Q_meas] -> First-Order Filter1/1
  Qref_pu/1 -> Sum4/2
  Sum5/1 -> Vd_ref/1
  Constant/1 -> Vq_ref/1

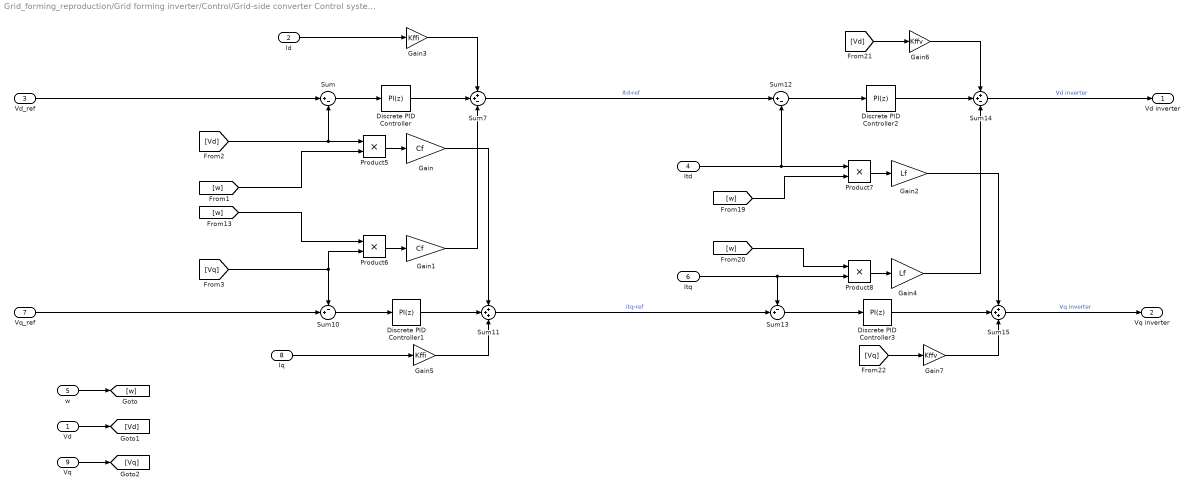
== system Grid_forming_reproduction/Grid forming inverter/Control/Grid-side converter Control system/Subsystem/Inner loops ==
  Vd : Inport
  Id : Inport  Port=2
  Vd_ref : Inport  Port=3
  Itd : Inport  Port=4
  w : Inport  Port=5
  Itq : Inport  Port=6
  Vq_ref : Inport  Port=7
  Iq : Inport  Port=8
  Vq : Inport  Port=9
  Discrete PID Controller : slpidlib/PID Controller  Controller=PI  Form=Parallel  TimeDomain=Discrete-time  UseExternalTs=off  SampleTime=Ts  IntegratorMethod=Forward Euler  FilterMethod=Forward Euler  ControllerParametersSource=internal  P=Kp_vc  I=Ki_vc  UseKiTs=off  D=0  N=100  UseFilter=on  TunerSelectOption=Transfer Function Based (PID Tuner App)  InitialConditionSource=internal  InitialConditionForIntegrator=0  InitialConditionForFilter=0  DifferentiatorICPrevScaledInput=0  ExternalReset=none  TrackingMode=off  Kt=1  LimitOutput=off  SatLimitsSource=internal  UpperSaturationLimit=inf  LowerSaturationLimit=-inf  LinearizeAsGain=off  AntiWindupMode=none  Kb=1  LimitIntegrator=off  UpperIntegratorSaturationLimit=inf  LowerIntegratorSaturationLimit=-inf  POutMin=[]  POutMax=[]  IOutMin=[]  IOutMax=[]  DOutMin=[]  DOutMax=[]  NOutMin=[]  NOutMax=[]  SumOutMin=[]  SumOutMax=[]  SaturationOutMin=[]  SaturationOutMax=[]  PParamMin=[]  PParamMax=[]  IParamMin=[]  IParamMax=[]  DParamMin=[]  DParamMax=[]  NParamMin=[]  NParamMax=[]  KbParamMin=[]  KbParamMax=[]  KtParamMin=[]  KtParamMax=[]  KbOutMin=[]  KbOutMax=[]  KtOutMin=[]  KtOutMax=[]  IntegratorOutMin=[]  IntegratorOutMax=[]  FilterOutMin=[]  FilterOutMax=[]  SumI1OutMin=[]  SumI1OutMax=[]  SumI2OutMin=[]  SumI2OutMax=[]  SumI3OutMin=[]  SumI3OutMax=[]  SumI4OutMin=[]  SumI4OutMax=[]  SumDOutMin=[]  SumDOutMax=[]  DifferentiatorOutMin=[]  DifferentiatorOutMax=[]  FilterDiffOutCoefMin=[]  FilterDiffOutCoefMax=[]  ReciprocalOutMin=[]  ReciprocalOutMax=[]  SumDenOutMin=[]  SumDenOutMax=[]  SumNumOutMin=[]  SumNumOutMax=[]  DivideOutMin=[]  DivideOutMax=[]  UdiffTsProdOutMin=[]  UdiffTsProdOutMax=[]  NTsProdOutMin=[]  NTsProdOutMax=[]  UintegralTsProdOutMin=[]  UintegralTsProdOutMax=[]  UngainTsProdOutMin=[]  UngainTsProdOutMax=[]  ClampingZeroOutDataTypeStr=Inherit: Inherit via back propagation  ClampingZeroOutMin=[]  ClampingZeroOutMax=[]  FilterDenConstantOutDataTypeStr=Inherit: Inherit via back propagation  FilterDenConstantOutMin=[]  FilterDenConstantOutMax=[]  PCopyOutDataTypeStr=Inherit: Inherit via back propagation  PCopyOutMin=[]  PCopyOutMax=[]  NCopyOutDataTypeStr=Inherit: Inherit via back propagation  NCopyOutMin=[]  NCopyOutMax=[]  IntegratorContinuousStateAttributes=''  IntegratorStateMustResolveToSignalObject=off  IntegratorRTWStateStorageClass=Auto  FilterContinuousStateAttributes=''  FilterStateMustResolveToSignalObject=off  FilterRTWStateStorageClass=Auto  ParallelPVariant=InternalParameters  IdealPVariant=Disabled  IVariant=InternalParameters  DVariant=Disabled  IntegratorVariant=Discrete  SatVariant=Disabled  AWVariant=Passthrough  PCopyVariant=Disabled  TRVariant=Disabled  FdbkBlocksVariant=Forward  IdealPFdbkVariant=Disabled  SatFdbkVariant=Disabled  DerivativeFilterVariant=Disabled  NVariant=Disabled  NCopyVariant=Disabled_SignalSpec  FilterICVariant=Disabled  IntegratorICVariant=InternalICs  ExternalResetVariant=Disabled  TRSumVariant=Passthrough  SumFdbkVariant=Disabled  SumVariant=Sum_PI  TsampFilterVariant=InternalTs  TsampNgainVariant=Passthrough  TsampIntegralVariant=Disabled_SignalSpec  ExternalSaturationOutDataTypeStr=Inherit: Same as second input
  Discrete PID Controller1 : slpidlib/PID Controller  Controller=PI  Form=Parallel  TimeDomain=Discrete-time  UseExternalTs=off  SampleTime=Ts  IntegratorMethod=Forward Euler  FilterMethod=Forward Euler  ControllerParametersSource=internal  P=Kp_vc  I=Ki_vc  UseKiTs=off  D=0  N=100  UseFilter=on  TunerSelectOption=Transfer Function Based (PID Tuner App)  InitialConditionSource=internal  InitialConditionForIntegrator=0  InitialConditionForFilter=0  DifferentiatorICPrevScaledInput=0  ExternalReset=none  TrackingMode=off  Kt=1  LimitOutput=off  SatLimitsSource=internal  UpperSaturationLimit=inf  LowerSaturationLimit=-inf  LinearizeAsGain=off  AntiWindupMode=none  Kb=1  LimitIntegrator=off  UpperIntegratorSaturationLimit=inf  LowerIntegratorSaturationLimit=-inf  POutMin=[]  POutMax=[]  IOutMin=[]  IOutMax=[]  DOutMin=[]  DOutMax=[]  NOutMin=[]  NOutMax=[]  SumOutMin=[]  SumOutMax=[]  SaturationOutMin=[]  SaturationOutMax=[]  PParamMin=[]  PParamMax=[]  IParamMin=[]  IParamMax=[]  DParamMin=[]  DParamMax=[]  NParamMin=[]  NParamMax=[]  KbParamMin=[]  KbParamMax=[]  KtParamMin=[]  KtParamMax=[]  KbOutMin=[]  KbOutMax=[]  KtOutMin=[]  KtOutMax=[]  IntegratorOutMin=[]  IntegratorOutMax=[]  FilterOutMin=[]  FilterOutMax=[]  SumI1OutMin=[]  SumI1OutMax=[]  SumI2OutMin=[]  SumI2OutMax=[]  SumI3OutMin=[]  SumI3OutMax=[]  SumI4OutMin=[]  SumI4OutMax=[]  SumDOutMin=[]  SumDOutMax=[]  DifferentiatorOutMin=[]  DifferentiatorOutMax=[]  FilterDiffOutCoefMin=[]  FilterDiffOutCoefMax=[]  ReciprocalOutMin=[]  ReciprocalOutMax=[]  SumDenOutMin=[]  SumDenOutMax=[]  SumNumOutMin=[]  SumNumOutMax=[]  DivideOutMin=[]  DivideOutMax=[]  UdiffTsProdOutMin=[]  UdiffTsProdOutMax=[]  NTsProdOutMin=[]  NTsProdOutMax=[]  UintegralTsProdOutMin=[]  UintegralTsProdOutMax=[]  UngainTsProdOutMin=[]  UngainTsProdOutMax=[]  ClampingZeroOutDataTypeStr=Inherit: Inherit via back propagation  ClampingZeroOutMin=[]  ClampingZeroOutMax=[]  FilterDenConstantOutDataTypeStr=Inherit: Inherit via back propagation  FilterDenConstantOutMin=[]  FilterDenConstantOutMax=[]  PCopyOutDataTypeStr=Inherit: Inherit via back propagation  PCopyOutMin=[]  PCopyOutMax=[]  NCopyOutDataTypeStr=Inherit: Inherit via back propagation  NCopyOutMin=[]  NCopyOutMax=[]  IntegratorContinuousStateAttributes=''  IntegratorStateMustResolveToSignalObject=off  IntegratorRTWStateStorageClass=Auto  FilterContinuousStateAttributes=''  FilterStateMustResolveToSignalObject=off  FilterRTWStateStorageClass=Auto  ParallelPVariant=InternalParameters  IdealPVariant=Disabled  IVariant=InternalParameters  DVariant=Disabled  IntegratorVariant=Discrete  SatVariant=Disabled  AWVariant=Passthrough  PCopyVariant=Disabled  TRVariant=Disabled  FdbkBlocksVariant=Forward  IdealPFdbkVariant=Disabled  SatFdbkVariant=Disabled  DerivativeFilterVariant=Disabled  NVariant=Disabled  NCopyVariant=Disabled_SignalSpec  FilterICVariant=Disabled  IntegratorICVariant=InternalICs  ExternalResetVariant=Disabled  TRSumVariant=Passthrough  SumFdbkVariant=Disabled  SumVariant=Sum_PI  TsampFilterVariant=InternalTs  TsampNgainVariant=Passthrough  TsampIntegralVariant=Disabled_SignalSpec  ExternalSaturationOutDataTypeStr=Inherit: Same as second input
  Discrete PID Controller2 : slpidlib/PID Controller  Controller=PI  Form=Parallel  TimeDomain=Discrete-time  UseExternalTs=off  SampleTime=Ts  IntegratorMethod=Forward Euler  FilterMethod=Forward Euler  ControllerParametersSource=internal  P=Kp_cc  I=Ki_cc  UseKiTs=off  D=0  N=100  UseFilter=on  TunerSelectOption=Transfer Function Based (PID Tuner App)  InitialConditionSource=internal  InitialConditionForIntegrator=0  InitialConditionForFilter=0  DifferentiatorICPrevScaledInput=0  ExternalReset=none  TrackingMode=off  Kt=1  LimitOutput=off  SatLimitsSource=internal  UpperSaturationLimit=inf  LowerSaturationLimit=-inf  LinearizeAsGain=off  AntiWindupMode=none  Kb=1  LimitIntegrator=off  UpperIntegratorSaturationLimit=inf  LowerIntegratorSaturationLimit=-inf  POutMin=[]  POutMax=[]  IOutMin=[]  IOutMax=[]  DOutMin=[]  DOutMax=[]  NOutMin=[]  NOutMax=[]  SumOutMin=[]  SumOutMax=[]  SaturationOutMin=[]  SaturationOutMax=[]  PParamMin=[]  PParamMax=[]  IParamMin=[]  IParamMax=[]  DParamMin=[]  DParamMax=[]  NParamMin=[]  NParamMax=[]  KbParamMin=[]  KbParamMax=[]  KtParamMin=[]  KtParamMax=[]  KbOutMin=[]  KbOutMax=[]  KtOutMin=[]  KtOutMax=[]  IntegratorOutMin=[]  IntegratorOutMax=[]  FilterOutMin=[]  FilterOutMax=[]  SumI1OutMin=[]  SumI1OutMax=[]  SumI2OutMin=[]  SumI2OutMax=[]  SumI3OutMin=[]  SumI3OutMax=[]  SumI4OutMin=[]  SumI4OutMax=[]  SumDOutMin=[]  SumDOutMax=[]  DifferentiatorOutMin=[]  DifferentiatorOutMax=[]  FilterDiffOutCoefMin=[]  FilterDiffOutCoefMax=[]  ReciprocalOutMin=[]  ReciprocalOutMax=[]  SumDenOutMin=[]  SumDenOutMax=[]  SumNumOutMin=[]  SumNumOutMax=[]  DivideOutMin=[]  DivideOutMax=[]  UdiffTsProdOutMin=[]  UdiffTsProdOutMax=[]  NTsProdOutMin=[]  NTsProdOutMax=[]  UintegralTsProdOutMin=[]  UintegralTsProdOutMax=[]  UngainTsProdOutMin=[]  UngainTsProdOutMax=[]  ClampingZeroOutDataTypeStr=Inherit: Inherit via back propagation  ClampingZeroOutMin=[]  ClampingZeroOutMax=[]  FilterDenConstantOutDataTypeStr=Inherit: Inherit via back propagation  FilterDenConstantOutMin=[]  FilterDenConstantOutMax=[]  PCopyOutDataTypeStr=Inherit: Inherit via back propagation  PCopyOutMin=[]  PCopyOutMax=[]  NCopyOutDataTypeStr=Inherit: Inherit via back propagation  NCopyOutMin=[]  NCopyOutMax=[]  IntegratorContinuousStateAttributes=''  IntegratorStateMustResolveToSignalObject=off  IntegratorRTWStateStorageClass=Auto  FilterContinuousStateAttributes=''  FilterStateMustResolveToSignalObject=off  FilterRTWStateStorageClass=Auto  ParallelPVariant=InternalParameters  IdealPVariant=Disabled  IVariant=InternalParameters  DVariant=Disabled  IntegratorVariant=Discrete  SatVariant=Disabled  AWVariant=Passthrough  PCopyVariant=Disabled  TRVariant=Disabled  FdbkBlocksVariant=Forward  IdealPFdbkVariant=Disabled  SatFdbkVariant=Disabled  DerivativeFilterVariant=Disabled  NVariant=Disabled  NCopyVariant=Disabled_SignalSpec  FilterICVariant=Disabled  IntegratorICVariant=InternalICs  ExternalResetVariant=Disabled  TRSumVariant=Passthrough  SumFdbkVariant=Disabled  SumVariant=Sum_PI  TsampFilterVariant=InternalTs  TsampNgainVariant=Passthrough  TsampIntegralVariant=Disabled_SignalSpec  ExternalSaturationOutDataTypeStr=Inherit: Same as second input
  Discrete PID Controller3 : slpidlib/PID Controller  Controller=PI  Form=Parallel  TimeDomain=Discrete-time  UseExternalTs=off  SampleTime=Ts  IntegratorMethod=Forward Euler  FilterMethod=Forward Euler  ControllerParametersSource=internal  P=Kp_cc  I=Ki_cc  UseKiTs=off  D=0  N=100  UseFilter=on  TunerSelectOption=Transfer Function Based (PID Tuner App)  InitialConditionSource=internal  InitialConditionForIntegrator=0  InitialConditionForFilter=0  DifferentiatorICPrevScaledInput=0  ExternalReset=none  TrackingMode=off  Kt=1  LimitOutput=off  SatLimitsSource=internal  UpperSaturationLimit=inf  LowerSaturationLimit=-inf  LinearizeAsGain=off  AntiWindupMode=none  Kb=1  LimitIntegrator=off  UpperIntegratorSaturationLimit=inf  LowerIntegratorSaturationLimit=-inf  POutMin=[]  POutMax=[]  IOutMin=[]  IOutMax=[]  DOutMin=[]  DOutMax=[]  NOutMin=[]  NOutMax=[]  SumOutMin=[]  SumOutMax=[]  SaturationOutMin=[]  SaturationOutMax=[]  PParamMin=[]  PParamMax=[]  IParamMin=[]  IParamMax=[]  DParamMin=[]  DParamMax=[]  NParamMin=[]  NParamMax=[]  KbParamMin=[]  KbParamMax=[]  KtParamMin=[]  KtParamMax=[]  KbOutMin=[]  KbOutMax=[]  KtOutMin=[]  KtOutMax=[]  IntegratorOutMin=[]  IntegratorOutMax=[]  FilterOutMin=[]  FilterOutMax=[]  SumI1OutMin=[]  SumI1OutMax=[]  SumI2OutMin=[]  SumI2OutMax=[]  SumI3OutMin=[]  SumI3OutMax=[]  SumI4OutMin=[]  SumI4OutMax=[]  SumDOutMin=[]  SumDOutMax=[]  DifferentiatorOutMin=[]  DifferentiatorOutMax=[]  FilterDiffOutCoefMin=[]  FilterDiffOutCoefMax=[]  ReciprocalOutMin=[]  ReciprocalOutMax=[]  SumDenOutMin=[]  SumDenOutMax=[]  SumNumOutMin=[]  SumNumOutMax=[]  DivideOutMin=[]  DivideOutMax=[]  UdiffTsProdOutMin=[]  UdiffTsProdOutMax=[]  NTsProdOutMin=[]  NTsProdOutMax=[]  UintegralTsProdOutMin=[]  UintegralTsProdOutMax=[]  UngainTsProdOutMin=[]  UngainTsProdOutMax=[]  ClampingZeroOutDataTypeStr=Inherit: Inherit via back propagation  ClampingZeroOutMin=[]  ClampingZeroOutMax=[]  FilterDenConstantOutDataTypeStr=Inherit: Inherit via back propagation  FilterDenConstantOutMin=[]  FilterDenConstantOutMax=[]  PCopyOutDataTypeStr=Inherit: Inherit via back propagation  PCopyOutMin=[]  PCopyOutMax=[]  NCopyOutDataTypeStr=Inherit: Inherit via back propagation  NCopyOutMin=[]  NCopyOutMax=[]  IntegratorContinuousStateAttributes=''  IntegratorStateMustResolveToSignalObject=off  IntegratorRTWStateStorageClass=Auto  FilterContinuousStateAttributes=''  FilterStateMustResolveToSignalObject=off  FilterRTWStateStorageClass=Auto  ParallelPVariant=InternalParameters  IdealPVariant=Disabled  IVariant=InternalParameters  DVariant=Disabled  IntegratorVariant=Discrete  SatVariant=Disabled  AWVariant=Passthrough  PCopyVariant=Disabled  TRVariant=Disabled  FdbkBlocksVariant=Forward  IdealPFdbkVariant=Disabled  SatFdbkVariant=Disabled  DerivativeFilterVariant=Disabled  NVariant=Disabled  NCopyVariant=Disabled_SignalSpec  FilterICVariant=Disabled  IntegratorICVariant=InternalICs  ExternalResetVariant=Disabled  TRSumVariant=Passthrough  SumFdbkVariant=Disabled  SumVariant=Sum_PI  TsampFilterVariant=InternalTs  TsampNgainVariant=Passthrough  TsampIntegralVariant=Disabled_SignalSpec  ExternalSaturationOutDataTypeStr=Inherit: Same as second input
  Gain : Gain  Gain=Cf
  Gain1 : Gain  Gain=Cf
  Gain2 : Gain  Gain=Lf
  Gain3 : Gain  Gain=Kffi
  Gain4 : Gain  Gain=Lf
  Gain5 : Gain  Gain=Kffi
  Gain6 : Gain  Gain=Kffv
  Gain7 : Gain  Gain=Kffv
  Product{5..8} (4 alike) : Product
  Sum : Sum  Inputs=|+-
  Sum10 : Sum  Inputs=-+|
  Sum11 : Sum  Inputs=+++
  Sum12 : Sum  Inputs=|+-
  Sum13 : Sum  Inputs=-+|
  Sum14 : Sum  Inputs=++-
  Sum15 : Sum  Inputs=+++
  Sum7 : Sum  Inputs=++-
  Vd inverter : Outport
  Vq inverter : Outport  Port=2
  wires:
  [Vq] -> Sum10/1, Product6/2
  Itd/1 -> Sum12/2, Product7/1
  Sum/1 -> Discrete PID Controller/1
  [w] -> Product8/1
  Iq/1 -> Gain5/1
  Sum11/1 -> Sum13/2  "itq-ref"
  Vd_ref/1 -> Sum/1
  [Vq] -> Gain7/1
  Gain2/1 -> Sum15/1
  [Vd] -> Gain6/1
  [Vd] -> Sum/2, Product5/1
  Sum7/1 -> Sum12/1  "Itd-ref"
  Product5/1 -> Gain/1
  [w] -> Product5/2
  Sum10/1 -> Discrete PID Controller1/1
  Gain3/1 -> Sum7/1
  Itq/1 -> Sum13/1, Product8/2
  Sum15/1 -> Vq inverter/1  "Vq inverter"
  [w] -> Product6/1
  Product6/1 -> Gain1/1
  Gain/1 -> Sum11/1
  [w] -> Product7/2
  Sum12/1 -> Discrete PID Controller2/1
  Vq_ref/1 -> Sum10/2
  Discrete PID Controller/1 -> Sum7/2
  Gain5/1 -> Sum11/3
  Gain4/1 -> Sum14/3
  Sum13/1 -> Discrete PID Controller3/1
  Gain1/1 -> Sum7/3
  Sum14/1 -> Vd inverter/1  "Vd inverter"
  Id/1 -> Gain3/1
  Product7/1 -> Gain2/1
  Product8/1 -> Gain4/1
  Discrete PID Controller2/1 -> Sum14/2
  Discrete PID Controller1/1 -> Sum11/2
  Gain6/1 -> Sum14/1
  Discrete PID Controller3/1 -> Sum15/2
  Gain7/1 -> Sum15/3
  w/1 -> [w]
  Vd/1 -> [Vd]
  Vq/1 -> [Vq]

== system Grid_forming_reproduction/Grid forming inverter/Control/Grid-side converter Control system/Subsystem/No inner loops ==
  Vd_ref : Inport
  Vq_ref : Inport  Port=2
  Vd inverter : Outport
  Vq inverter : Outport  Port=2
  wires:
  Vd_ref/1 -> Vd inverter/1
  Vq_ref/1 -> Vq inverter/1

== system Grid_forming_reproduction/Grid forming inverter/Control/Grid-side converter Control system/Virtual impedance/No virtual impedance ==
  Vd_ref : Inport
  Vq_ref : Inport  Port=2
  Vd_ref* : Outport
  Vq_ref* : Outport  Port=2
  wires:
  Vd_ref/1 -> Vd_ref*/1
  Vq_ref/1 -> Vq_ref*/1

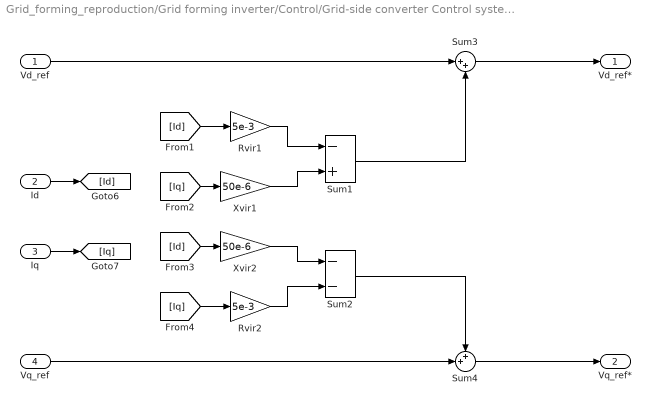
== system Grid_forming_reproduction/Grid forming inverter/Control/Grid-side converter Control system/Virtual impedance/Virtual impedance ==
  Vd_ref : Inport
  Id : Inport  Port=2
  Iq : Inport  Port=3
  Vq_ref : Inport  Port=4
  Rvir1 : Gain  Gain=5e-3
  Rvir2 : Gain  Gain=5e-3
  Sum1 : Sum  Inputs=-+
  Sum2 : Sum  Inputs=--
  Sum3 : Sum  Inputs=|++
  Sum4 : Sum  Inputs=++|
  Xvir1 : Gain  Gain=50e-6
  Xvir2 : Gain  Gain=50e-6
  Vd_ref* : Outport
  Vq_ref* : Outport  Port=2
  wires:
  Sum2/1 -> Sum4/1
  Xvir1/1 -> Sum1/2
  Sum1/1 -> Sum3/2
  Sum3/1 -> Vd_ref*/1
  Rvir2/1 -> Sum2/2
  Xvir2/1 -> Sum2/1
  Rvir1/1 -> Sum1/1
  [Iq] -> Xvir1/1
  [Id] -> Xvir2/1
  Vq_ref/1 -> Sum4/2
  Sum4/1 -> Vq_ref*/1
  [Id] -> Rvir1/1
  [Iq] -> Rvir2/1
  Vd_ref/1 -> Sum3/1
  Id/1 -> [Id]
  Iq/1 -> [Iq]
